simulink model "Microcontroller"  (R2026a)
settings: Solver=FixedStepDiscrete  StopTime=120  FixedStep=p.Ts
InitFcn:
  | cartpole_system_init
undefined symbols (not defined in the file): Kd_aug, Ld, p, x0_phys
settings Model: Creator=david  LastModifiedBy=david
settings HardwareCC: ProdLargestAtomicInteger=Long  ProdLargestAtomicFloat=Double  ProdHWDeviceType=ARM Compatible->ARM Cortex-M
settings RTWCC: SystemTargetFile=ert.tlc  Description=Embedded Coder
settings ERTTargetCC: GenerateSampleERTMain=on
settings ExplorerConfigSet: InternalSimMechanicsExplorerSettings=|
  | <ExplorerConfiguration>
  | 
  |   <canonicalview>default</canonicalview>
  | 
  |   <TilePanel>
  |     <TileInfo>
  |       <Tiles Columns="1" Count="1" Height="610" Rows="1" Width="1536">
  |         <Row Weight="1"/>
  |         <Column Weight="1"/>
  |         <Tile Height="1" Width="1" X="0" Y="0"/>
  |       </Tiles>
  |     </TileInfo>
  |     <SceneInfo>
  |       <SceneViewer>
  |         <IsThisViewStd>
  |           <IsStandardView>off</IsStandardView>
  |           <StandardViewName>Front</StandardViewName>
  |         </IsThisViewStd>
  |         <BGColor>
  |           <R>1</R>
  |           <G>1</G>
  |           <B>1</B>
  |           <A>1</A>
  |         </BGColor>
  |         <Camera>
  |           <DoPerspective>off</DoPerspective>
  |           <Position>
  |             <X>-0.38733030516761002</X>
  |             <Y>0.60926147831297028</Y>
  |             <Z>3.3549500429517707</Z>
  |           </Position>
  |           <Center>
  |             <X>-0.38733030516761002</X>
  |             <Y>0.60926147831297028</Y>
  |             <Z>-0.019999999403953556</Z>
  |           </Center>
  |           <Up>
  |             <X>0</X>
  |             <Y>1</Y>
  |             <Z>0</Z>
  |           </Up>
  |           <XLim>1.3855356409800417</XLim>
  |           <YLim>1.3855356409800417</YLim>
  |           <ViewLimDist>0.01</ViewLimDist>
  |         </Camera>
  |       </SceneViewer>
  |     </SceneInfo>
  |   </TilePanel>
  | 
  |   <MechEditorPanel>
  |     <GfxPanelCameraMap/>
  |     <Cameras/>
  |     <VideoCreator>
  |       <IncludeTiles>All</IncludeTiles>
  |       <IncludeTime>on</IncludeTime>
  |       <IncludeWorldFrame>off</IncludeWorldFrame>
  |       <PlaybackSpeedRatio>1</PlaybackSpeedRatio>
  |       <FrameRate>30</FrameRate>
  |       <FrameSize>auto</FrameSize>
  |       <VideoFormat>UncompressedAVI</VideoFormat>
  |     </VideoCreator>
  |   </MechEditorPanel>
  | 
  |   <PlaybackSettings>
  |     <PlaybackSpeedFactor>8</PlaybackSpeedFactor>
  |   </PlaybackSettings>
  | 
  | </ExplorerConfiguration>

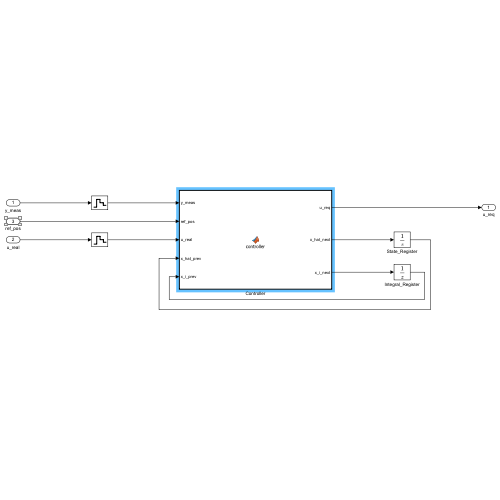
[thumbnail: Simulink's stored preview of the top-level diagram]
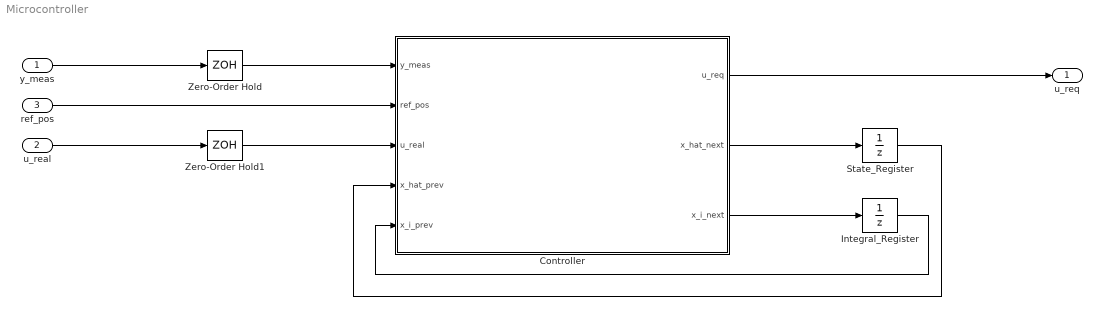
== system Microcontroller ==
  y_meas : Inport  OutDataTypeStr=single  PortDimensions=2
  u_real : Inport  Port=2  OutDataTypeStr=single  PortDimensions=1
  ref_pos : Inport  Port=3  OutDataTypeStr=single  PortDimensions=1
  Controller : MATLAB Function  TreatAsAtomicUnit=on
  Integral_Register : UnitDelay  InitialCondition=single(0)  SampleTime=p.Ts
  State_Register : UnitDelay  InitialCondition=single(x0_phys)  SampleTime=p.Ts
  Zero-Order Hold : ZeroOrderHold  SampleTime=p.Ts
  Zero-Order Hold1 : ZeroOrderHold  SampleTime=p.Ts
  u_req : Outport  OutDataTypeStr=single  PortDimensions=1
  wires:
  y_meas/1 -> Zero-Order Hold/1
  Controller/1(u_req) -> u_req/1
  u_real/1 -> Zero-Order Hold1/1
  Zero-Order Hold/1 -> Controller/1(y_meas)
  ref_pos/1 -> Controller/2(ref_pos)
  Controller/2(x_hat_next) -> State_Register/1
  Controller/3(x_i_next) -> Integral_Register/1
  State_Register/1 -> Controller/4(x_hat_prev)
  Integral_Register/1 -> Controller/5(x_i_prev)
  Zero-Order Hold1/1 -> Controller/3(u_real)

== matlab function Microcontroller/Controller ==
  data: y_meas input single; u_req output single; ref_pos input single; u_real input single; x_hat_prev input single; x_i_prev input single; x_hat_next output; x_i_next output; p parameter; Kd_aug parameter; Ld parameter
function [u_req, x_hat_next, x_i_next] = controller(y_meas, ref_pos, u_real, x_hat_prev, x_i_prev, p, Kd_aug, Ld)
    x_hat_cart = x_hat_prev(1);
    dx_hat     = x_hat_prev(2);
    th_hat     = x_hat_prev(3);
    dth_hat    = x_hat_prev(4);
    
    th_err_lqi = atan2(sin(th_hat), cos(th_hat));
    
    x_lqi = [x_hat_cart - ref_pos; dx_hat; th_err_lqi; dth_hat];
    
    N_approx_est  = compute_normal_force_approx(th_hat, dth_hat, p);
    F_coulomb_est = p.mu_c * N_approx_est;
    u_ff = p.ff_compensation * F_coulomb_est * tanh(p.k * dx_hat);
    
    u_lqi = -Kd_aug(1:4) * x_lqi - Kd_aug(5) * x_i_prev;
    
    E_kinetic   = 0.5 * p.m * (p.l * dth_hat)^2;
    E_potential = p.m * p.g * p.l * cos(th_hat); 
    E_current   = E_kinetic + E_potential;
    E_target    = p.m * p.g * p.l;
    E_error     = E_current - E_target;

    x_penalty = p.swing.k_p * ((x_hat_cart - ref_pos) / p.TRACK_LIMIT)^3;
    
    is_down_and_still = exp(-0.5 * (dth_hat/0.2)^2) * exp(-0.5 * ((cos(th_hat) + 1)/0.05)^2);
    u_kick = p.swing.kick_amp * is_down_and_still;
    
    u_swing = p.swing.k_E * E_error * dth_hat * cos(th_hat) - x_penalty - p.swing.k_d * dx_hat + u_kick;
    
    sigma = p.swing.th_thresh / 1.5; 
    weight_LQI = exp(-0.5 * (abs(th_err_lqi) / sigma)^6);
    u_req_unclamped = weight_LQI * u_lqi + (1 - weight_LQI) * u_swing + u_ff;
    
    error_i = weight_LQI * (y_meas(1) - ref_pos);
    
    if (u_req_unclamped >= p.U_MAX && error_i > 0) || (u_req_unclamped <= -p.U_MAX && error_i < 0)
        dx_i = single(0); 
    else
        dx_i = error_i;
    end
    
    x_i_next = x_i_prev + p.Ts * dx_i;
    u_req = max(min(u_req_unclamped, p.U_MAX), -p.U_MAX);
    
    F_ext_hat = 0;
    M_ext_hat = 0;
    
    q_ddot_est = compute_accelerations(dx_hat, th_hat, dth_hat, u_real, p, F_ext_hat, M_ext_hat);
    
    f_x_hat = [dx_hat; q_ddot_est(1); dth_hat; q_ddot_est(2)];
    
    y_hat = [x_hat_cart; th_hat];
    residual_raw = y_meas - y_hat;
    
    innovation = [residual_raw(1); 
                  atan2(sin(residual_raw(2)), cos(residual_raw(2)))];
                  
    x_hat_next = x_hat_prev + p.Ts * f_x_hat + Ld * innovation;
end
